simulink model "latest_coil"  (R2021b)
settings: Solver=FixedStepAuto  StartTime=-18e-3  StopTime=50e-3  FixedStep=1e-4  RelTol=1e-3
undefined symbols (not defined in the file): X, Y, Z
libraries: sm_lib x28, nesl_utility x9
(part 3 of 5)

== matlab function latest_coil/Inner Coil/Coil 1/FIELD Y ==
  data: X input; Hx_yp output; Y input; Z input; I input; Hy_yp output; Hz_yp output; Hx_yn output; Hy_yn output; Hz_yn output; dBx_dx output; dBx_dy output; dBx_dz output; dBz_dx output; dBz_dy output; dBz_dz output
function [Hx_yp, Hy_yp, Hz_yp, Hx_yn, Hy_yn, Hz_yn, dBx_dx, dBx_dy, dBx_dz, dBz_dx, dBz_dy, dBz_dz] = field_y(X, Y, Z, I)

n = 1;
gy = 520e-6;
% gx = 675e-6;
gz = 0;
m0 = 4*pi*1e-7;
k = 0.4e-3;
yp1 = -0.6e-3 - (n-1)*k;
yp2 = 0.6e-3 + (n-1)*k;
a_xp = gy;
a_zp = gz;
k_yp = 1./(4*pi*((a_xp-X).^2+(a_zp-Z).^2));
kyp = (yp2-Y)./((yp2-Y).^2+(a_xp-X).^2+(a_zp-Z).^2).^0.5;
k_2yp = (yp1-Y)./((yp1-Y).^2+(a_xp-X).^2+(a_zp-Z).^2).^0.5;

Hx_yp = -((a_zp-Z).*k_yp.*(kyp - k_2yp))*I*m0;
Hy_yp = zeros(size(X,1),size(Y,1),size(Z,1));
Hz_yp = (-(a_xp-X).*k_yp.*(kyp - k_2yp))*I*m0;

a_xn = -gy;
yn1 = -0.8e-3 - (n-1)*k;
yn2 = 0.8e-3 + (n-1)*k;
k_yn = 1./(4*pi*((a_xn-X).^2+(a_zp-Z).^2));
kyn = (yn2-Y)./((yn2-Y).^2+(a_xn-X).^2+(a_zp-Z).^2).^0.5;
k_2yn = (yn1-Y)./((yn1-Y).^2+(a_xn-X).^2+(a_zp-Z).^2).^0.5;

Hx_yn = ((a_zp-Z).*k_yn.*(kyn - k_2yn))*I*m0;
Hy_yn = zeros(size(X,1),size(Y,1),size(Z,1));
Hz_yn = ((a_xn-X).*k_yn.*(kyn - k_2yn))*I*m0;


dBxn_dx = - (I*Z*m0*(((Y - yn1)*(2*X - 2*a_xn))/(2*((X - a_xn)^2 + (Z - a_zp)^2 + (Y - yn1)^2)^(3/2)) - ((Y - yn2)*(2*X - 2*a_xn))/(2*((X - a_xn)^2 + (Z - a_zp)^2 + (Y - yn2)^2)^(3/2))))/(4*pi*((X - a_xn)^2 + (Z - a_zp)^2)) - (I*Z*m0*((Y - yn1)/((X - a_xn)^2 + (Z - a_zp)^2 + (Y - yn1)^2)^(1/2) - (Y - yn2)/((X - a_xn)^2 + (Z - a_zp)^2 + (Y - yn2)^2)^(1/2))*(2*X - 2*a_xn))/(4*pi*((X - a_xn)^2 + (Z - a_zp)^2)^2);
dBxp_dx = (I*Z*m0*(((Y - yp1)*(2*X - 2*a_xp))/(2*((X - a_xp)^2 + (Z - a_zp)^2 + (Y - yp1)^2)^(3/2)) - ((Y - yp2)*(2*X - 2*a_xp))/(2*((X - a_xp)^2 + (Z - a_zp)^2 + (Y - yp2)^2)^(3/2))))/(4*pi*((X - a_xp)^2 + (Z - a_zp)^2)) + (I*Z*m0*((Y - yp1)/((X - a_xp)^2 + (Z - a_zp)^2 + (Y - yp1)^2)^(1/2) - (Y - yp2)/((X - a_xp)^2 + (Z - a_zp)^2 + (Y - yp2)^2)^(1/2))*(2*X - 2*a_xp))/(4*pi*((X - a_xp)^2 + (Z - a_zp)^2)^2);
dBx_dx = dBxp_dx + dBxn_dx;

dBxp_dy = -(I*Z*m0*(1/((X - a_xp)^2 + (Z - a_zp)^2 + (Y - yp1)^2)^(1/2) - 1/((X - a_xp)^2 + (Z - a_zp)^2 + (Y - yp2)^2)^(1/2) - ((Y - yp1)*(2*Y - 2*yp1))/(2*((X - a_xp)^2 + (Z - a_zp)^2 + (Y - yp1)^2)^(3/2)) + ((Y - yp2)*(2*Y - 2*yp2))/(2*((X - a_xp)^2 + (Z - a_zp)^2 + (Y - yp2)^2)^(3/2))))/(4*pi*((X - a_xp)^2 + (Z - a_zp)^2));
dBxn_dy = (I*Z*m0*(1/((X - a_xn)^2 + (Z - a_zp)^2 + (Y - yn1)^2)^(1/2) - 1/((X - a_xn)^2 + (Z - a_zp)^2 + (Y - yn2)^2)^(1/2) - ((Y - yn1)*(2*Y - 2*yn1))/(2*((X - a_xn)^2 + (Z - a_zp)^2 + (Y - yn1)^2)^(3/2)) + ((Y - yn2)*(2*Y - 2*yn2))/(2*((X - a_xn)^2 + (Z - a_zp)^2 + (Y - yn2)^2)^(3/2))))/(4*pi*((X - a_xn)^2 + (Z - a_zp)^2));
dBx_dy = dBxp_dy + dBxn_dy;

dBxp_dz = (I*Z*m0*(((Y - yp1)*(2*Z - 2*a_zp))/(2*((X - a_xp)^2 + (Z - a_zp)^2 + (Y - yp1)^2)^(3/2)) - ((Y - yp2)*(2*Z - 2*a_zp))/(2*((X - a_xp)^2 + (Z - a_zp)^2 + (Y - yp2)^2)^(3/2))))/(4*pi*((X - a_xp)^2 + (Z - a_zp)^2)) - (I*m0*((Y - yp1)/((X - a_xp)^2 + (Z - a_zp)^2 + (Y - yp1)^2)^(1/2) - (Y - yp2)/((X - a_xp)^2 + (Z - a_zp)^2 + (Y - yp2)^2)^(1/2)))/(4*pi*((X - a_xp)^2 + (Z - a_zp)^2)) + (I*Z*m0*((Y - yp1)/((X - a_xp)^2 + (Z - a_zp)^2 + (Y - yp1)^2)^(1/2) - (Y - yp2)/((X - a_xp)^2 + (Z - a_zp)^2 + (Y - yp2)^2)^(1/2))*(2*Z - 2*a_zp))/(4*pi*((X - a_xp)^2 + (Z - a_zp)^2)^2);
dBxn_dz = (I*m0*((Y - yn1)/((X - a_xn)^2 + (Z - a_zp)^2 + (Y - yn1)^2)^(1/2) - (Y - yn2)/((X - a_xn)^2 + (Z - a_zp)^2 + (Y - yn2)^2)^(1/2)))/(4*pi*((X - a_xn)^2 + (Z - a_zp)^2)) - (I*Z*m0*(((Y - yn1)*(2*Z - 2*a_zp))/(2*((X - a_xn)^2 + (Z - a_zp)^2 + (Y - yn1)^2)^(3/2)) - ((Y - yn2)*(2*Z - 2*a_zp))/(2*((X - a_xn)^2 + (Z - a_zp)^2 + (Y - yn2)^2)^(3/2))))/(4*pi*((X - a_xn)^2 + (Z - a_zp)^2)) - (I*Z*m0*((Y - yn1)/((X - a_xn)^2 + (Z - a_zp)^2 + (Y - yn1)^2)^(1/2) - (Y - yn2)/((X - a_xn)^2 + (Z - a_zp)^2 + (Y - yn2)^2)^(1/2))*(2*Z - 2*a_zp))/(4*pi*((X - a_xn)^2 + (Z - a_zp)^2)^2);
dBx_dz = dBxp_dz + dBxn_dz;

dBzn_dx = (I*m0*(X - a_xn)*(((Y - yn1)*(2*X - 2*a_xn))/(2*((X - a_xn)^2 + (Z - a_zp)^2 + (Y - yn1)^2)^(3/2)) - ((Y - yn2)*(2*X - 2*a_xn))/(2*((X - a_xn)^2 + (Z - a_zp)^2 + (Y - yn2)^2)^(3/2))))/(4*pi*(Z^2 + (X - a_xn)^2)) - (I*m0*((Y - yn1)/((X - a_xn)^2 + (Z - a_zp)^2 + (Y - yn1)^2)^(1/2) - (Y - yn2)/((X - a_xn)^2 + (Z - a_zp)^2 + (Y - yn2)^2)^(1/2)))/(4*pi*(Z^2 + (X - a_xn)^2)) + (I*m0*((Y - yn1)/((X - a_xn)^2 + (Z - a_zp)^2 + (Y - yn1)^2)^(1/2) - (Y - yn2)/((X - a_xn)^2 + (Z - a_zp)^2 + (Y - yn2)^2)^(1/2))*(X - a_xn)*(2*X - 2*a_xn))/(4*pi*(Z^2 + (X - a_xn)^2)^2);
dBzp_dx = (I*m0*((Y - yp1)/((X - a_xp)^2 + (Z - a_zp)^2 + (Y - yp1)^2)^(1/2) - (Y - yp2)/((X - a_xp)^2 + (Z - a_zp)^2 + (Y - yp2)^2)^(1/2)))/(4*pi*(Z^2 + (X - a_xp)^2)) - (I*m0*(X - a_xp)*(((Y - yp1)*(2*X - 2*a_xp))/(2*((X - a_xp)^2 + (Z - a_zp)^2 + (Y - yp1)^2)^(3/2)) - ((Y - yp2)*(2*X - 2*a_xp))/(2*((X - a_xp)^2 + (Z - a_zp)^2 + (Y - yp2)^2)^(3/2))))/(4*pi*(Z^2 + (X - a_xp)^2)) - (I*m0*((Y - yp1)/((X - a_xp)^2 + (Z - a_zp)^2 + (Y - yp1)^2)^(1/2) - (Y - yp2)/((X - a_xp)^2 + (Z - a_zp)^2 + (Y - yp2)^2)^(1/2))*(X - a_xp)*(2*X - 2*a_xp))/(4*pi*(Z^2 + (X - a_xp)^2)^2);
dBz_dx = dBzp_dx + dBzn_dx;

dBzn_dy = -(I*m0*(X - a_xn)*(1/((X - a_xn)^2 + (Z - a_zp)^2 + (Y - yn1)^2)^(1/2) - 1/((X - a_xn)^2 + (Z - a_zp)^2 + (Y - yn2)^2)^(1/2) - ((Y - yn1)*(2*Y - 2*yn1))/(2*((X - a_xn)^2 + (Z - a_zp)^2 + (Y - yn1)^2)^(3/2)) + ((Y - yn2)*(2*Y - 2*yn2))/(2*((X - a_xn)^2 + (Z - a_zp)^2 + (Y - yn2)^2)^(3/2))))/(4*pi*(Z^2 + (X - a_xn)^2));
dBzp_dy = (I*m0*(X - a_xp)*(1/((X - a_xp)^2 + (Z - a_zp)^2 + (Y - yp1)^2)^(1/2) - 1/((X - a_xp)^2 + (Z - a_zp)^2 + (Y - yp2)^2)^(1/2) - ((Y - yp1)*(2*Y - 2*yp1))/(2*((X - a_xp)^2 + (Z - a_zp)^2 + (Y - yp1)^2)^(3/2)) + ((Y - yp2)*(2*Y - 2*yp2))/(2*((X - a_xp)^2 + (Z - a_zp)^2 + (Y - yp2)^2)^(3/2))))/(4*pi*(Z^2 + (X - a_xp)^2));
dBz_dy = dBzn_dy + dBzp_dy;

dBzn_dz = (I*m0*(X - a_xn)*(((Y - yn1)*(2*Z - 2*a_zp))/(2*((X - a_xn)^2 + (Z - a_zp)^2 + (Y - yn1)^2)^(3/2)) - ((Y - yn2)*(2*Z - 2*a_zp))/(2*((X - a_xn)^2 + (Z - a_zp)^2 + (Y - yn2)^2)^(3/2))))/(4*pi*(Z^2 + (X - a_xn)^2)) + (I*Z*m0*((Y - yn1)/((X - a_xn)^2 + (Z - a_zp)^2 + (Y - yn1)^2)^(1/2) - (Y - yn2)/((X - a_xn)^2 + (Z - a_zp)^2 + (Y - yn2)^2)^(1/2))*(X - a_xn))/(2*pi*(Z^2 + (X - a_xn)^2)^2);
dBzp_dz = - (I*m0*(X - a_xp)*(((Y - yp1)*(2*Z - 2*a_zp))/(2*((X - a_xp)^2 + (Z - a_zp)^2 + (Y - yp1)^2)^(3/2)) - ((Y - yp2)*(2*Z - 2*a_zp))/(2*((X - a_xp)^2 + (Z - a_zp)^2 + (Y - yp2)^2)^(3/2))))/(4*pi*(Z^2 + (X - a_xp)^2)) - (I*Z*m0*((Y - yp1)/((X - a_xp)^2 + (Z - a_zp)^2 + (Y - yp1)^2)^(1/2) - (Y - yp2)/((X - a_xp)^2 + (Z - a_zp)^2 + (Y - yp2)^2)^(1/2))*(X - a_xp))/(2*pi*(Z^2 + (X - a_xp)^2)^2);
dBz_dz = dBzn_dz + dBzp_dz;
end

== matlab function latest_coil/Inner Coil/Coil 5/MATLAB Function ==
  data: X input; Hx_xp output; Y input; Z input; I input; Hy_xp output; Hz_xp output; Hx_xn output; Hy_xn output; Hz_xn output; dBy_dx output; dBy_dy output; dBy_dz output; dBz_dx output; dBz_dy output; dBz_dz output
function [Hx_xp, Hy_xp, Hz_xp, Hx_xn, Hy_xn, Hz_xn,dBy_dx ,dBy_dy, dBy_dz, dBz_dx ,dBz_dy, dBz_dz] = field_x(X, Y, Z, I)
n = 5;
gy = 424e-6;
gx = 2.275e-3;
gz = 0;
m0 = 4*pi*1e-7;
k = 0.4e-3;
xp1 = -0.8e-3 - (n-1)*k;
xp2 = 0.8e-3 + (n-1)*k;
a_yp = gx; 
a_zp = gz;
k_p = 1./(4*pi*((a_yp-Y).^2+(a_zp-Z).^2));
kxp = (xp2-X)./((xp2-X).^2+(a_yp-Y).^2+(a_zp-Z).^2).^0.5;
k_2xp = (xp1-X)./((xp1-X).^2+(a_yp-Y).^2+(a_zp-Z).^2).^0.5;

Hx_xp = zeros(size(X,1),size(Y,1),size(Z,1));
Hy_xp = (-(a_zp-Z).*k_p.*(kxp - k_2xp))*I*m0;
Hz_xp = (-(a_yp-Y).*k_p.*(kxp - k_2xp))*I*m0;

a_yn = -gx;
xn1 = -1e-3 - (n-1)*k;
xn2 = 1e-3 + (n-1)*k;
k_n = 1./(4*pi*((a_yn-Y).^2+(a_zp-Z).^2));
kxn = (xn2-X)./((xn2-X).^2+(a_yn-Y).^2+(a_zp-Z).^2).^0.5;
k_2xn = (xn1-X)./((xn1-X).^2+(a_yn-Y).^2+(a_zp-Z).^2).^0.5;

Hx_xn = zeros(size(X,1),size(Y,1),size(Z,1));
Hy_xn = ((a_zp-Z).*k_n.*(kxn - k_2xn))*I*m0;
Hz_xn = ((a_yn-Y).*k_n.*(kxn - k_2xn))*I*m0;

dByn_dx = (I*Z*m0*(1/((Y - a_yn)^2 + (Z - a_zp)^2 + (X - xn1)^2)^(1/2) - 1/((Y - a_yn)^2 + (Z - a_zp)^2 + (X - xn2)^2)^(1/2) - ((X - xn1)*(2*X - 2*xn1))/(2*((Y - a_yn)^2 + (Z - a_zp)^2 + (X - xn1)^2)^(3/2)) + ((X - xn2)*(2*X - 2*xn2))/(2*((Y - a_yn)^2 + (Z - a_zp)^2 + (X - xn2)^2)^(3/2))))/(4*pi*((Y - a_yn)^2 + (Z - a_zp)^2));
dByp_dx = -(I*Z*m0*(1/((Y - a_yp)^2 + (Z - a_zp)^2 + (X - xp1)^2)^(1/2) - 1/((Y - a_yp)^2 + (Z - a_zp)^2 + (X - xp2)^2)^(1/2) - ((X - xp1)*(2*X - 2*xp1))/(2*((Y - a_yp)^2 + (Z - a_zp)^2 + (X - xp1)^2)^(3/2)) + ((X - xp2)*(2*X - 2*xp2))/(2*((Y - a_yp)^2 + (Z - a_zp)^2 + (X - xp2)^2)^(3/2))))/(4*pi*((Y - a_yp)^2 + (Z - a_zp)^2));
dBy_dx = dByp_dx + dByn_dx;

dByp_dy = (I*Z*m0*(((X - xp1)*(2*Y - 2*a_yp))/(2*((Y - a_yp)^2 + (Z - a_zp)^2 + (X - xp1)^2)^(3/2)) - ((X - xp2)*(2*Y - 2*a_yp))/(2*((Y - a_yp)^2 + (Z - a_zp)^2 + (X - xp2)^2)^(3/2))))/(4*pi*((Y - a_yp)^2 + (Z - a_zp)^2)) + (I*Z*m0*(2*Y - 2*a_yp)*((X - xp1)/((Y - a_yp)^2 + (Z - a_zp)^2 + (X - xp1)^2)^(1/2) - (X - xp2)/((Y - a_yp)^2 + (Z - a_zp)^2 + (X - xp2)^2)^(1/2)))/(4*pi*((Y - a_yp)^2 + (Z - a_zp)^2)^2);
dByn_dy = - (I*Z*m0*(((X - xn1)*(2*Y - 2*a_yn))/(2*((Y - a_yn)^2 + (Z - a_zp)^2 + (X - xn1)^2)^(3/2)) - ((X - xn2)*(2*Y - 2*a_yn))/(2*((Y - a_yn)^2 + (Z - a_zp)^2 + (X - xn2)^2)^(3/2))))/(4*pi*((Y - a_yn)^2 + (Z - a_zp)^2)) - (I*Z*m0*(2*Y - 2*a_yn)*((X - xn1)/((Y - a_yn)^2 + (Z - a_zp)^2 + (X - xn1)^2)^(1/2) - (X - xn2)/((Y - a_yn)^2 + (Z - a_zp)^2 + (X - xn2)^2)^(1/2)))/(4*pi*((Y - a_yn)^2 + (Z - a_zp)^2)^2);
dBy_dy = dByp_dy + dByn_dy;

dByp_dz = (I*Z*m0*(((X - xp1)*(2*Z - 2*a_zp))/(2*((Y - a_yp)^2 + (Z - a_zp)^2 + (X - xp1)^2)^(3/2)) - ((X - xp2)*(2*Z - 2*a_zp))/(2*((Y - a_yp)^2 + (Z - a_zp)^2 + (X - xp2)^2)^(3/2))))/(4*pi*((Y - a_yp)^2 + (Z - a_zp)^2)) - (I*m0*((X - xp1)/((Y - a_yp)^2 + (Z - a_zp)^2 + (X - xp1)^2)^(1/2) - (X - xp2)/((Y - a_yp)^2 + (Z - a_zp)^2 + (X - xp2)^2)^(1/2)))/(4*pi*((Y - a_yp)^2 + (Z - a_zp)^2)) + (I*Z*m0*(2*Z - 2*a_zp)*((X - xp1)/((Y - a_yp)^2 + (Z - a_zp)^2 + (X - xp1)^2)^(1/2) - (X - xp2)/((Y - a_yp)^2 + (Z - a_zp)^2 + (X - xp2)^2)^(1/2)))/(4*pi*((Y - a_yp)^2 + (Z - a_zp)^2)^2);
dByn_dz = (I*m0*((X - xn1)/((Y - a_yn)^2 + (Z - a_zp)^2 + (X - xn1)^2)^(1/2) - (X - xn2)/((Y - a_yn)^2 + (Z - a_zp)^2 + (X - xn2)^2)^(1/2)))/(4*pi*((Y - a_yn)^2 + (Z - a_zp)^2)) - (I*Z*m0*(((X - xn1)*(2*Z - 2*a_zp))/(2*((Y - a_yn)^2 + (Z - a_zp)^2 + (X - xn1)^2)^(3/2)) - ((X - xn2)*(2*Z - 2*a_zp))/(2*((Y - a_yn)^2 + (Z - a_zp)^2 + (X - xn2)^2)^(3/2))))/(4*pi*((Y - a_yn)^2 + (Z - a_zp)^2)) - (I*Z*m0*(2*Z - 2*a_zp)*((X - xn1)/((Y - a_yn)^2 + (Z - a_zp)^2 + (X - xn1)^2)^(1/2) - (X - xn2)/((Y - a_yn)^2 + (Z - a_zp)^2 + (X - xn2)^2)^(1/2)))/(4*pi*((Y - a_yn)^2 + (Z - a_zp)^2)^2);
dBy_dz = dByp_dz + dByn_dz;

dBzp_dx = (I*m0*(Y - a_yp)*(1/((Y - a_yp)^2 + (Z - a_zp)^2 + (X - xp1)^2)^(1/2) - 1/((Y - a_yp)^2 + (Z - a_zp)^2 + (X - xp2)^2)^(1/2) - ((X - xp1)*(2*X - 2*xp1))/(2*((Y - a_yp)^2 + (Z - a_zp)^2 + (X - xp1)^2)^(3/2)) + ((X - xp2)*(2*X - 2*xp2))/(2*((Y - a_yp)^2 + (Z - a_zp)^2 + (X - xp2)^2)^(3/2))))/(4*pi*(Z^2 + (Y - a_yp)^2));
dBzn_dx = -(I*m0*(Y - a_yn)*(1/((Y - a_yn)^2 + (Z - a_zp)^2 + (X - xn1)^2)^(1/2) - 1/((Y - a_yn)^2 + (Z - a_zp)^2 + (X - xn2)^2)^(1/2) - ((X - xn1)*(2*X - 2*xn1))/(2*((Y - a_yn)^2 + (Z - a_zp)^2 + (X - xn1)^2)^(3/2)) + ((X - xn2)*(2*X - 2*xn2))/(2*((Y - a_yn)^2 + (Z - a_zp)^2 + (X - xn2)^2)^(3/2))))/(4*pi*(Z^2 + (Y - a_yn)^2));
dBz_dx = dBzp_dx + dBzn_dx;

dBzn_dy = (I*m0*(Y - a_yn)*(((X - xn1)*(2*Y - 2*a_yn))/(2*((Y - a_yn)^2 + (Z - a_zp)^2 + (X - xn1)^2)^(3/2)) - ((X - xn2)*(2*Y - 2*a_yn))/(2*((Y - a_yn)^2 + (Z - a_zp)^2 + (X - xn2)^2)^(3/2))))/(4*pi*(Z^2 + (Y - a_yn)^2)) - (I*m0*((X - xn1)/((Y - a_yn)^2 + (Z - a_zp)^2 + (X - xn1)^2)^(1/2) - (X - xn2)/((Y - a_yn)^2 + (Z - a_zp)^2 + (X - xn2)^2)^(1/2)))/(4*pi*(Z^2 + (Y - a_yn)^2)) + (I*m0*(Y - a_yn)*(2*Y - 2*a_yn)*((X - xn1)/((Y - a_yn)^2 + (Z - a_zp)^2 + (X - xn1)^2)^(1/2) - (X - xn2)/((Y - a_yn)^2 + (Z - a_zp)^2 + (X - xn2)^2)^(1/2)))/(4*pi*(Z^2 + (Y - a_yn)^2)^2);
dBzp_dy = (I*m0*((X - xp1)/((Y - a_yp)^2 + (Z - a_zp)^2 + (X - xp1)^2)^(1/2) - (X - xp2)/((Y - a_yp)^2 + (Z - a_zp)^2 + (X - xp2)^2)^(1/2)))/(4*pi*(Z^2 + (Y - a_yp)^2)) - (I*m0*(Y - a_yp)*(((X - xp1)*(2*Y - 2*a_yp))/(2*((Y - a_yp)^2 + (Z - a_zp)^2 + (X - xp1)^2)^(3/2)) - ((X - xp2)*(2*Y - 2*a_yp))/(2*((Y - a_yp)^2 + (Z - a_zp)^2 + (X - xp2)^2)^(3/2))))/(4*pi*(Z^2 + (Y - a_yp)^2)) - (I*m0*(Y - a_yp)*(2*Y - 2*a_yp)*((X - xp1)/((Y - a_yp)^2 + (Z - a_zp)^2 + (X - xp1)^2)^(1/2) - (X - xp2)/((Y - a_yp)^2 + (Z - a_zp)^2 + (X - xp2)^2)^(1/2)))/(4*pi*(Z^2 + (Y - a_yp)^2)^2);
dBz_dy = dBzn_dy + dBzp_dy;

dBzn_dz = (I*m0*(Y - a_yn)*(((X - xn1)*(2*Z - 2*a_zp))/(2*((Y - a_yn)^2 + (Z - a_zp)^2 + (X - xn1)^2)^(3/2)) - ((X - xn2)*(2*Z - 2*a_zp))/(2*((Y - a_yn)^2 + (Z - a_zp)^2 + (X - xn2)^2)^(3/2))))/(4*pi*(Z^2 + (Y - a_yn)^2)) + (I*Z*m0*(Y - a_yn)*((X - xn1)/((Y - a_yn)^2 + (Z - a_zp)^2 + (X - xn1)^2)^(1/2) - (X - xn2)/((Y - a_yn)^2 + (Z - a_zp)^2 + (X - xn2)^2)^(1/2)))/(2*pi*(Z^2 + (Y - a_yn)^2)^2);
dBzp_dz = - (I*m0*(Y - a_yp)*(((X - xp1)*(2*Z - 2*a_zp))/(2*((Y - a_yp)^2 + (Z - a_zp)^2 + (X - xp1)^2)^(3/2)) - ((X - xp2)*(2*Z - 2*a_zp))/(2*((Y - a_yp)^2 + (Z - a_zp)^2 + (X - xp2)^2)^(3/2))))/(4*pi*(Z^2 + (Y - a_yp)^2)) - (I*Z*m0*(Y - a_yp)*((X - xp1)/((Y - a_yp)^2 + (Z - a_zp)^2 + (X - xp1)^2)^(1/2) - (X - xp2)/((Y - a_yp)^2 + (Z - a_zp)^2 + (X - xp2)^2)^(1/2)))/(2*pi*(Z^2 + (Y - a_yp)^2)^2);
dBz_dz = dBzn_dz + dBzp_dz;
end

== matlab function latest_coil/Inner Coil/Coil 5/MATLAB Function3 ==
  data: X input; Hx_yp output; Y input; Z input; I input; Hy_yp output; Hz_yp output; Hx_yn output; Hy_yn output; Hz_yn output; dBx_dx output; dBx_dy output; dBx_dz output; dBz_dx output; dBz_dy output; dBz_dz output
function [Hx_yp, Hy_yp, Hz_yp, Hx_yn, Hy_yn, Hz_yn, dBx_dx, dBx_dy, dBx_dz, dBz_dx, dBz_dy, dBz_dz] = field_y(X, Y, Z, I)
n = 5;
gy = 424e-6;
gx = 2.275e-3;
gz = 0;
m0 = 4*pi*1e-7;
k = 0.4e-3;
yp1 = -0.6e-3 - (n-1)*k;
yp2 = 0.6e-3 + (n-1)*k;
a_xp = gy;
a_zp = gz;
k_yp = 1./(4*pi*((a_xp-X).^2+(a_zp-Z).^2));
kyp = (yp2-Y)./((yp2-Y).^2+(a_xp-X).^2+(a_zp-Z).^2).^0.5;
k_2yp = (yp1-Y)./((yp1-Y).^2+(a_xp-X).^2+(a_zp-Z).^2).^0.5;

Hx_yp = -((a_zp-Z).*k_yp.*(kyp - k_2yp))*I*m0;
Hy_yp = zeros(size(X,1),size(Y,1),size(Z,1));
Hz_yp = (-(a_xp-X).*k_yp.*(kyp - k_2yp))*I*m0;

a_xn = -gy;
yn1 = -0.8e-3 - (n-1)*k;
yn2 = 0.8e-3 + (n-1)*k;
k_yn = 1./(4*pi*((a_xn-X).^2+(a_zp-Z).^2));
kyn = (yn2-Y)./((yn2-Y).^2+(a_xn-X).^2+(a_zp-Z).^2).^0.5;
k_2yn = (yn1-Y)./((yn1-Y).^2+(a_xn-X).^2+(a_zp-Z).^2).^0.5;

Hx_yn = ((a_zp-Z).*k_yn.*(kyn - k_2yn))*I*m0;
Hy_yn = zeros(size(X,1),size(Y,1),size(Z,1));
Hz_yn = ((a_xn-X).*k_yn.*(kyn - k_2yn))*I*m0;

dBxn_dx = - (I*Z*m0*(((Y - yn1)*(2*X - 2*a_xn))/(2*((X - a_xn)^2 + (Z - a_zp)^2 + (Y - yn1)^2)^(3/2)) - ((Y - yn2)*(2*X - 2*a_xn))/(2*((X - a_xn)^2 + (Z - a_zp)^2 + (Y - yn2)^2)^(3/2))))/(4*pi*((X - a_xn)^2 + (Z - a_zp)^2)) - (I*Z*m0*((Y - yn1)/((X - a_xn)^2 + (Z - a_zp)^2 + (Y - yn1)^2)^(1/2) - (Y - yn2)/((X - a_xn)^2 + (Z - a_zp)^2 + (Y - yn2)^2)^(1/2))*(2*X - 2*a_xn))/(4*pi*((X - a_xn)^2 + (Z - a_zp)^2)^2);
dBxp_dx = (I*Z*m0*(((Y - yp1)*(2*X - 2*a_xp))/(2*((X - a_xp)^2 + (Z - a_zp)^2 + (Y - yp1)^2)^(3/2)) - ((Y - yp2)*(2*X - 2*a_xp))/(2*((X - a_xp)^2 + (Z - a_zp)^2 + (Y - yp2)^2)^(3/2))))/(4*pi*((X - a_xp)^2 + (Z - a_zp)^2)) + (I*Z*m0*((Y - yp1)/((X - a_xp)^2 + (Z - a_zp)^2 + (Y - yp1)^2)^(1/2) - (Y - yp2)/((X - a_xp)^2 + (Z - a_zp)^2 + (Y - yp2)^2)^(1/2))*(2*X - 2*a_xp))/(4*pi*((X - a_xp)^2 + (Z - a_zp)^2)^2);
dBx_dx = dBxp_dx + dBxn_dx;

dBxp_dy = -(I*Z*m0*(1/((X - a_xp)^2 + (Z - a_zp)^2 + (Y - yp1)^2)^(1/2) - 1/((X - a_xp)^2 + (Z - a_zp)^2 + (Y - yp2)^2)^(1/2) - ((Y - yp1)*(2*Y - 2*yp1))/(2*((X - a_xp)^2 + (Z - a_zp)^2 + (Y - yp1)^2)^(3/2)) + ((Y - yp2)*(2*Y - 2*yp2))/(2*((X - a_xp)^2 + (Z - a_zp)^2 + (Y - yp2)^2)^(3/2))))/(4*pi*((X - a_xp)^2 + (Z - a_zp)^2));
dBxn_dy = (I*Z*m0*(1/((X - a_xn)^2 + (Z - a_zp)^2 + (Y - yn1)^2)^(1/2) - 1/((X - a_xn)^2 + (Z - a_zp)^2 + (Y - yn2)^2)^(1/2) - ((Y - yn1)*(2*Y - 2*yn1))/(2*((X - a_xn)^2 + (Z - a_zp)^2 + (Y - yn1)^2)^(3/2)) + ((Y - yn2)*(2*Y - 2*yn2))/(2*((X - a_xn)^2 + (Z - a_zp)^2 + (Y - yn2)^2)^(3/2))))/(4*pi*((X - a_xn)^2 + (Z - a_zp)^2));
dBx_dy = dBxp_dy + dBxn_dy;

dBxp_dz = (I*Z*m0*(((Y - yp1)*(2*Z - 2*a_zp))/(2*((X - a_xp)^2 + (Z - a_zp)^2 + (Y - yp1)^2)^(3/2)) - ((Y - yp2)*(2*Z - 2*a_zp))/(2*((X - a_xp)^2 + (Z - a_zp)^2 + (Y - yp2)^2)^(3/2))))/(4*pi*((X - a_xp)^2 + (Z - a_zp)^2)) - (I*m0*((Y - yp1)/((X - a_xp)^2 + (Z - a_zp)^2 + (Y - yp1)^2)^(1/2) - (Y - yp2)/((X - a_xp)^2 + (Z - a_zp)^2 + (Y - yp2)^2)^(1/2)))/(4*pi*((X - a_xp)^2 + (Z - a_zp)^2)) + (I*Z*m0*((Y - yp1)/((X - a_xp)^2 + (Z - a_zp)^2 + (Y - yp1)^2)^(1/2) - (Y - yp2)/((X - a_xp)^2 + (Z - a_zp)^2 + (Y - yp2)^2)^(1/2))*(2*Z - 2*a_zp))/(4*pi*((X - a_xp)^2 + (Z - a_zp)^2)^2);
dBxn_dz = (I*m0*((Y - yn1)/((X - a_xn)^2 + (Z - a_zp)^2 + (Y - yn1)^2)^(1/2) - (Y - yn2)/((X - a_xn)^2 + (Z - a_zp)^2 + (Y - yn2)^2)^(1/2)))/(4*pi*((X - a_xn)^2 + (Z - a_zp)^2)) - (I*Z*m0*(((Y - yn1)*(2*Z - 2*a_zp))/(2*((X - a_xn)^2 + (Z - a_zp)^2 + (Y - yn1)^2)^(3/2)) - ((Y - yn2)*(2*Z - 2*a_zp))/(2*((X - a_xn)^2 + (Z - a_zp)^2 + (Y - yn2)^2)^(3/2))))/(4*pi*((X - a_xn)^2 + (Z - a_zp)^2)) - (I*Z*m0*((Y - yn1)/((X - a_xn)^2 + (Z - a_zp)^2 + (Y - yn1)^2)^(1/2) - (Y - yn2)/((X - a_xn)^2 + (Z - a_zp)^2 + (Y - yn2)^2)^(1/2))*(2*Z - 2*a_zp))/(4*pi*((X - a_xn)^2 + (Z - a_zp)^2)^2);
dBx_dz = dBxp_dz + dBxn_dz;

dBzn_dx = (I*m0*(X - a_xn)*(((Y - yn1)*(2*X - 2*a_xn))/(2*((X - a_xn)^2 + (Z - a_zp)^2 + (Y - yn1)^2)^(3/2)) - ((Y - yn2)*(2*X - 2*a_xn))/(2*((X - a_xn)^2 + (Z - a_zp)^2 + (Y - yn2)^2)^(3/2))))/(4*pi*(Z^2 + (X - a_xn)^2)) - (I*m0*((Y - yn1)/((X - a_xn)^2 + (Z - a_zp)^2 + (Y - yn1)^2)^(1/2) - (Y - yn2)/((X - a_xn)^2 + (Z - a_zp)^2 + (Y - yn2)^2)^(1/2)))/(4*pi*(Z^2 + (X - a_xn)^2)) + (I*m0*((Y - yn1)/((X - a_xn)^2 + (Z - a_zp)^2 + (Y - yn1)^2)^(1/2) - (Y - yn2)/((X - a_xn)^2 + (Z - a_zp)^2 + (Y - yn2)^2)^(1/2))*(X - a_xn)*(2*X - 2*a_xn))/(4*pi*(Z^2 + (X - a_xn)^2)^2);
dBzp_dx = (I*m0*((Y - yp1)/((X - a_xp)^2 + (Z - a_zp)^2 + (Y - yp1)^2)^(1/2) - (Y - yp2)/((X - a_xp)^2 + (Z - a_zp)^2 + (Y - yp2)^2)^(1/2)))/(4*pi*(Z^2 + (X - a_xp)^2)) - (I*m0*(X - a_xp)*(((Y - yp1)*(2*X - 2*a_xp))/(2*((X - a_xp)^2 + (Z - a_zp)^2 + (Y - yp1)^2)^(3/2)) - ((Y - yp2)*(2*X - 2*a_xp))/(2*((X - a_xp)^2 + (Z - a_zp)^2 + (Y - yp2)^2)^(3/2))))/(4*pi*(Z^2 + (X - a_xp)^2)) - (I*m0*((Y - yp1)/((X - a_xp)^2 + (Z - a_zp)^2 + (Y - yp1)^2)^(1/2) - (Y - yp2)/((X - a_xp)^2 + (Z - a_zp)^2 + (Y - yp2)^2)^(1/2))*(X - a_xp)*(2*X - 2*a_xp))/(4*pi*(Z^2 + (X - a_xp)^2)^2);
dBz_dx = dBzp_dx + dBzn_dx;

dBzn_dy = -(I*m0*(X - a_xn)*(1/((X - a_xn)^2 + (Z - a_zp)^2 + (Y - yn1)^2)^(1/2) - 1/((X - a_xn)^2 + (Z - a_zp)^2 + (Y - yn2)^2)^(1/2) - ((Y - yn1)*(2*Y - 2*yn1))/(2*((X - a_xn)^2 + (Z - a_zp)^2 + (Y - yn1)^2)^(3/2)) + ((Y - yn2)*(2*Y - 2*yn2))/(2*((X - a_xn)^2 + (Z - a_zp)^2 + (Y - yn2)^2)^(3/2))))/(4*pi*(Z^2 + (X - a_xn)^2));
dBzp_dy = (I*m0*(X - a_xp)*(1/((X - a_xp)^2 + (Z - a_zp)^2 + (Y - yp1)^2)^(1/2) - 1/((X - a_xp)^2 + (Z - a_zp)^2 + (Y - yp2)^2)^(1/2) - ((Y - yp1)*(2*Y - 2*yp1))/(2*((X - a_xp)^2 + (Z - a_zp)^2 + (Y - yp1)^2)^(3/2)) + ((Y - yp2)*(2*Y - 2*yp2))/(2*((X - a_xp)^2 + (Z - a_zp)^2 + (Y - yp2)^2)^(3/2))))/(4*pi*(Z^2 + (X - a_xp)^2));
dBz_dy = dBzn_dy + dBzp_dy;

dBzn_dz = (I*m0*(X - a_xn)*(((Y - yn1)*(2*Z - 2*a_zp))/(2*((X - a_xn)^2 + (Z - a_zp)^2 + (Y - yn1)^2)^(3/2)) - ((Y - yn2)*(2*Z - 2*a_zp))/(2*((X - a_xn)^2 + (Z - a_zp)^2 + (Y - yn2)^2)^(3/2))))/(4*pi*(Z^2 + (X - a_xn)^2)) + (I*Z*m0*((Y - yn1)/((X - a_xn)^2 + (Z - a_zp)^2 + (Y - yn1)^2)^(1/2) - (Y - yn2)/((X - a_xn)^2 + (Z - a_zp)^2 + (Y - yn2)^2)^(1/2))*(X - a_xn))/(2*pi*(Z^2 + (X - a_xn)^2)^2);
dBzp_dz = - (I*m0*(X - a_xp)*(((Y - yp1)*(2*Z - 2*a_zp))/(2*((X - a_xp)^2 + (Z - a_zp)^2 + (Y - yp1)^2)^(3/2)) - ((Y - yp2)*(2*Z - 2*a_zp))/(2*((X - a_xp)^2 + (Z - a_zp)^2 + (Y - yp2)^2)^(3/2))))/(4*pi*(Z^2 + (X - a_xp)^2)) - (I*Z*m0*((Y - yp1)/((X - a_xp)^2 + (Z - a_zp)^2 + (Y - yp1)^2)^(1/2) - (Y - yp2)/((X - a_xp)^2 + (Z - a_zp)^2 + (Y - yp2)^2)^(1/2))*(X - a_xp))/(2*pi*(Z^2 + (X - a_xp)^2)^2);
dBz_dz = dBzn_dz + dBzp_dz;
end

== matlab function latest_coil/Inner Coil/Coil 5/MATLAB Function4 ==
  data: Hx_xp input; Hy_xp input; Hz_xp input; Hx output; Hx_xn input; Hy_xn input; Hy output; Hz output; Hz_xn input; Hx_yp input; Hy_yp input; Hz_yp input; Hx_yn input; Hy_yn input; Hz_yn input
function [Hx, Hy, Hz] = field_sum(Hx_xp, Hy_xp, Hz_xp, Hx_xn, Hy_xn, Hz_xn, Hx_yp, Hy_yp, Hz_yp, Hx_yn, Hy_yn, Hz_yn)
Hx = Hx_xp + Hx_xn + Hx_yp + Hx_yn;
Hy = Hy_xp + Hy_xn + Hy_yp + Hy_yn;
Hz = Hz_xp + Hz_xn + Hz_yp + Hz_yn;
end

== matlab function latest_coil/Outer Coil/Coil 6/MATLAB Function ==
  data: X input; Hx_xp output; Y input; Z input; I input; Hy_xp output; Hz_xp output; Hx_xn output; Hy_xn output; Hz_xn output; dBy_dx output; dBy_dy output; dBy_dz output; dBz_dx output; dBz_dy output; dBz_dz output
function [Hx_xp, Hy_xp, Hz_xp, Hx_xn, Hy_xn, Hz_xn,dBy_dx ,dBy_dy, dBy_dz, dBz_dx ,dBz_dy, dBz_dz] = field_x(X, Y, Z, I)
n = 6;
% gy = 420e-6;
gx = 2.675e-3; 
gz = 0;
m0 = 4*pi*1e-7;
k = 0.4e-3;
xp1 = -0.8e-3 - (n-1)*k;
xp2 = 0.8e-3 + (n-1)*k;
a_yp = gx; 
a_zp = gz;
k_p = 1./(4*pi*((a_yp-Y).^2+(a_zp-Z).^2));
kxp = (xp2-X)./((xp2-X).^2+(a_yp-Y).^2+(a_zp-Z).^2).^0.5;
k_2xp = (xp1-X)./((xp1-X).^2+(a_yp-Y).^2+(a_zp-Z).^2).^0.5;

Hx_xp = zeros(size(X,1),size(Y,1),size(Z,1));
Hy_xp = (-(a_zp-Z).*k_p.*(kxp - k_2xp))*I*m0;
Hz_xp = (-(a_yp-Y).*k_p.*(kxp - k_2xp))*I*m0;

a_yn = -gx;
xn1 = -1e-3 - (n-1)*k;
xn2 = 1e-3 + (n-1)*k;
k_n = 1./(4*pi*((a_yn-Y).^2+(a_zp-Z).^2));
kxn = (xn2-X)./((xn2-X).^2+(a_yn-Y).^2+(a_zp-Z).^2).^0.5;
k_2xn = (xn1-X)./((xn1-X).^2+(a_yn-Y).^2+(a_zp-Z).^2).^0.5;

Hx_xn = zeros(size(X,1),size(Y,1),size(Z,1));
Hy_xn = ((a_zp-Z).*k_n.*(kxn - k_2xn))*I*m0;
Hz_xn = ((a_yn-Y).*k_n.*(kxn - k_2xn))*I*m0;
dByn_dx = (I*Z*m0*(1/((Y - a_yn)^2 + (Z - a_zp)^2 + (X - xn1)^2)^(1/2) - 1/((Y - a_yn)^2 + (Z - a_zp)^2 + (X - xn2)^2)^(1/2) - ((X - xn1)*(2*X - 2*xn1))/(2*((Y - a_yn)^2 + (Z - a_zp)^2 + (X - xn1)^2)^(3/2)) + ((X - xn2)*(2*X - 2*xn2))/(2*((Y - a_yn)^2 + (Z - a_zp)^2 + (X - xn2)^2)^(3/2))))/(4*pi*((Y - a_yn)^2 + (Z - a_zp)^2));
dByp_dx = -(I*Z*m0*(1/((Y - a_yp)^2 + (Z - a_zp)^2 + (X - xp1)^2)^(1/2) - 1/((Y - a_yp)^2 + (Z - a_zp)^2 + (X - xp2)^2)^(1/2) - ((X - xp1)*(2*X - 2*xp1))/(2*((Y - a_yp)^2 + (Z - a_zp)^2 + (X - xp1)^2)^(3/2)) + ((X - xp2)*(2*X - 2*xp2))/(2*((Y - a_yp)^2 + (Z - a_zp)^2 + (X - xp2)^2)^(3/2))))/(4*pi*((Y - a_yp)^2 + (Z - a_zp)^2));
dBy_dx = dByp_dx + dByn_dx;

dByp_dy = (I*Z*m0*(((X - xp1)*(2*Y - 2*a_yp))/(2*((Y - a_yp)^2 + (Z - a_zp)^2 + (X - xp1)^2)^(3/2)) - ((X - xp2)*(2*Y - 2*a_yp))/(2*((Y - a_yp)^2 + (Z - a_zp)^2 + (X - xp2)^2)^(3/2))))/(4*pi*((Y - a_yp)^2 + (Z - a_zp)^2)) + (I*Z*m0*(2*Y - 2*a_yp)*((X - xp1)/((Y - a_yp)^2 + (Z - a_zp)^2 + (X - xp1)^2)^(1/2) - (X - xp2)/((Y - a_yp)^2 + (Z - a_zp)^2 + (X - xp2)^2)^(1/2)))/(4*pi*((Y - a_yp)^2 + (Z - a_zp)^2)^2);
dByn_dy = - (I*Z*m0*(((X - xn1)*(2*Y - 2*a_yn))/(2*((Y - a_yn)^2 + (Z - a_zp)^2 + (X - xn1)^2)^(3/2)) - ((X - xn2)*(2*Y - 2*a_yn))/(2*((Y - a_yn)^2 + (Z - a_zp)^2 + (X - xn2)^2)^(3/2))))/(4*pi*((Y - a_yn)^2 + (Z - a_zp)^2)) - (I*Z*m0*(2*Y - 2*a_yn)*((X - xn1)/((Y - a_yn)^2 + (Z - a_zp)^2 + (X - xn1)^2)^(1/2) - (X - xn2)/((Y - a_yn)^2 + (Z - a_zp)^2 + (X - xn2)^2)^(1/2)))/(4*pi*((Y - a_yn)^2 + (Z - a_zp)^2)^2);
dBy_dy = dByp_dy + dByn_dy;

dByp_dz = (I*Z*m0*(((X - xp1)*(2*Z - 2*a_zp))/(2*((Y - a_yp)^2 + (Z - a_zp)^2 + (X - xp1)^2)^(3/2)) - ((X - xp2)*(2*Z - 2*a_zp))/(2*((Y - a_yp)^2 + (Z - a_zp)^2 + (X - xp2)^2)^(3/2))))/(4*pi*((Y - a_yp)^2 + (Z - a_zp)^2)) - (I*m0*((X - xp1)/((Y - a_yp)^2 + (Z - a_zp)^2 + (X - xp1)^2)^(1/2) - (X - xp2)/((Y - a_yp)^2 + (Z - a_zp)^2 + (X - xp2)^2)^(1/2)))/(4*pi*((Y - a_yp)^2 + (Z - a_zp)^2)) + (I*Z*m0*(2*Z - 2*a_zp)*((X - xp1)/((Y - a_yp)^2 + (Z - a_zp)^2 + (X - xp1)^2)^(1/2) - (X - xp2)/((Y - a_yp)^2 + (Z - a_zp)^2 + (X - xp2)^2)^(1/2)))/(4*pi*((Y - a_yp)^2 + (Z - a_zp)^2)^2);
dByn_dz = (I*m0*((X - xn1)/((Y - a_yn)^2 + (Z - a_zp)^2 + (X - xn1)^2)^(1/2) - (X - xn2)/((Y - a_yn)^2 + (Z - a_zp)^2 + (X - xn2)^2)^(1/2)))/(4*pi*((Y - a_yn)^2 + (Z - a_zp)^2)) - (I*Z*m0*(((X - xn1)*(2*Z - 2*a_zp))/(2*((Y - a_yn)^2 + (Z - a_zp)^2 + (X - xn1)^2)^(3/2)) - ((X - xn2)*(2*Z - 2*a_zp))/(2*((Y - a_yn)^2 + (Z - a_zp)^2 + (X - xn2)^2)^(3/2))))/(4*pi*((Y - a_yn)^2 + (Z - a_zp)^2)) - (I*Z*m0*(2*Z - 2*a_zp)*((X - xn1)/((Y - a_yn)^2 + (Z - a_zp)^2 + (X - xn1)^2)^(1/2) - (X - xn2)/((Y - a_yn)^2 + (Z - a_zp)^2 + (X - xn2)^2)^(1/2)))/(4*pi*((Y - a_yn)^2 + (Z - a_zp)^2)^2);
dBy_dz = dByp_dz + dByn_dz;

dBzp_dx = (I*m0*(Y - a_yp)*(1/((Y - a_yp)^2 + (Z - a_zp)^2 + (X - xp1)^2)^(1/2) - 1/((Y - a_yp)^2 + (Z - a_zp)^2 + (X - xp2)^2)^(1/2) - ((X - xp1)*(2*X - 2*xp1))/(2*((Y - a_yp)^2 + (Z - a_zp)^2 + (X - xp1)^2)^(3/2)) + ((X - xp2)*(2*X - 2*xp2))/(2*((Y - a_yp)^2 + (Z - a_zp)^2 + (X - xp2)^2)^(3/2))))/(4*pi*(Z^2 + (Y - a_yp)^2));
dBzn_dx = -(I*m0*(Y - a_yn)*(1/((Y - a_yn)^2 + (Z - a_zp)^2 + (X - xn1)^2)^(1/2) - 1/((Y - a_yn)^2 + (Z - a_zp)^2 + (X - xn2)^2)^(1/2) - ((X - xn1)*(2*X - 2*xn1))/(2*((Y - a_yn)^2 + (Z - a_zp)^2 + (X - xn1)^2)^(3/2)) + ((X - xn2)*(2*X - 2*xn2))/(2*((Y - a_yn)^2 + (Z - a_zp)^2 + (X - xn2)^2)^(3/2))))/(4*pi*(Z^2 + (Y - a_yn)^2));
dBz_dx = dBzp_dx + dBzn_dx;

dBzn_dy = (I*m0*(Y - a_yn)*(((X - xn1)*(2*Y - 2*a_yn))/(2*((Y - a_yn)^2 + (Z - a_zp)^2 + (X - xn1)^2)^(3/2)) - ((X - xn2)*(2*Y - 2*a_yn))/(2*((Y - a_yn)^2 + (Z - a_zp)^2 + (X - xn2)^2)^(3/2))))/(4*pi*(Z^2 + (Y - a_yn)^2)) - (I*m0*((X - xn1)/((Y - a_yn)^2 + (Z - a_zp)^2 + (X - xn1)^2)^(1/2) - (X - xn2)/((Y - a_yn)^2 + (Z - a_zp)^2 + (X - xn2)^2)^(1/2)))/(4*pi*(Z^2 + (Y - a_yn)^2)) + (I*m0*(Y - a_yn)*(2*Y - 2*a_yn)*((X - xn1)/((Y - a_yn)^2 + (Z - a_zp)^2 + (X - xn1)^2)^(1/2) - (X - xn2)/((Y - a_yn)^2 + (Z - a_zp)^2 + (X - xn2)^2)^(1/2)))/(4*pi*(Z^2 + (Y - a_yn)^2)^2);
dBzp_dy = (I*m0*((X - xp1)/((Y - a_yp)^2 + (Z - a_zp)^2 + (X - xp1)^2)^(1/2) - (X - xp2)/((Y - a_yp)^2 + (Z - a_zp)^2 + (X - xp2)^2)^(1/2)))/(4*pi*(Z^2 + (Y - a_yp)^2)) - (I*m0*(Y - a_yp)*(((X - xp1)*(2*Y - 2*a_yp))/(2*((Y - a_yp)^2 + (Z - a_zp)^2 + (X - xp1)^2)^(3/2)) - ((X - xp2)*(2*Y - 2*a_yp))/(2*((Y - a_yp)^2 + (Z - a_zp)^2 + (X - xp2)^2)^(3/2))))/(4*pi*(Z^2 + (Y - a_yp)^2)) - (I*m0*(Y - a_yp)*(2*Y - 2*a_yp)*((X - xp1)/((Y - a_yp)^2 + (Z - a_zp)^2 + (X - xp1)^2)^(1/2) - (X - xp2)/((Y - a_yp)^2 + (Z - a_zp)^2 + (X - xp2)^2)^(1/2)))/(4*pi*(Z^2 + (Y - a_yp)^2)^2);
dBz_dy = dBzn_dy + dBzp_dy;

dBzn_dz = (I*m0*(Y - a_yn)*(((X - xn1)*(2*Z - 2*a_zp))/(2*((Y - a_yn)^2 + (Z - a_zp)^2 + (X - xn1)^2)^(3/2)) - ((X - xn2)*(2*Z - 2*a_zp))/(2*((Y - a_yn)^2 + (Z - a_zp)^2 + (X - xn2)^2)^(3/2))))/(4*pi*(Z^2 + (Y - a_yn)^2)) + (I*Z*m0*(Y - a_yn)*((X - xn1)/((Y - a_yn)^2 + (Z - a_zp)^2 + (X - xn1)^2)^(1/2) - (X - xn2)/((Y - a_yn)^2 + (Z - a_zp)^2 + (X - xn2)^2)^(1/2)))/(2*pi*(Z^2 + (Y - a_yn)^2)^2);
dBzp_dz = - (I*m0*(Y - a_yp)*(((X - xp1)*(2*Z - 2*a_zp))/(2*((Y - a_yp)^2 + (Z - a_zp)^2 + (X - xp1)^2)^(3/2)) - ((X - xp2)*(2*Z - 2*a_zp))/(2*((Y - a_yp)^2 + (Z - a_zp)^2 + (X - xp2)^2)^(3/2))))/(4*pi*(Z^2 + (Y - a_yp)^2)) - (I*Z*m0*(Y - a_yp)*((X - xp1)/((Y - a_yp)^2 + (Z - a_zp)^2 + (X - xp1)^2)^(1/2) - (X - xp2)/((Y - a_yp)^2 + (Z - a_zp)^2 + (X - xp2)^2)^(1/2)))/(2*pi*(Z^2 + (Y - a_yp)^2)^2);
dBz_dz = dBzn_dz + dBzp_dz;
end

== matlab function latest_coil/Outer Coil/Coil 6/MATLAB Function3 ==
  data: X input; Hx_yp output; Y input; Z input; I input; Hy_yp output; Hz_yp output; Hx_yn output; Hy_yn output; Hz_yn output; dBx_dx output; dBx_dy output; dBx_dz output; dBz_dx output; dBz_dy output; dBz_dz output
function [Hx_yp, Hy_yp, Hz_yp, Hx_yn, Hy_yn, Hz_yn, dBx_dx, dBx_dy, dBx_dz, dBz_dx, dBz_dy, dBz_dz] = field_y(X, Y, Z, I)

n = 6;
gy = 420e-6;
% gx = 2.675e-3; 
gz = 0;
m0 = 4*pi*1e-7;
k = 0.4e-3;
yp1 = -0.6e-3 - (n-1)*k;
yp2 = 0.6e-3 + (n-1)*k;
a_xp = gy;
a_zp = gz;
k_yp = 1./(4*pi*((a_xp-X).^2+(a_zp-Z).^2));
kyp = (yp2-Y)./((yp2-Y).^2+(a_xp-X).^2+(a_zp-Z).^2).^0.5;
k_2yp = (yp1-Y)./((yp1-Y).^2+(a_xp-X).^2+(a_zp-Z).^2).^0.5;

Hx_yp = -((a_zp-Z).*k_yp.*(kyp - k_2yp))*I*m0;
Hy_yp = zeros(size(X,1),size(Y,1),size(Z,1));
Hz_yp = (-(a_xp-X).*k_yp.*(kyp - k_2yp))*I*m0;

a_xn = -gy;
yn1 = -0.8e-3 - (n-1)*k;
yn2 = 0.8e-3 + (n-1)*k;
k_yn = 1./(4*pi*((a_xn-X).^2+(a_zp-Z).^2));
kyn = (yn2-Y)./((yn2-Y).^2+(a_xn-X).^2+(a_zp-Z).^2).^0.5;
k_2yn = (yn1-Y)./((yn1-Y).^2+(a_xn-X).^2+(a_zp-Z).^2).^0.5;

Hx_yn = ((a_zp-Z).*k_yn.*(kyn - k_2yn))*I*m0;
Hy_yn = zeros(size(X,1),size(Y,1),size(Z,1));
Hz_yn = ((a_xn-X).*k_yn.*(kyn - k_2yn))*I*m0;

dBxn_dx = - (I*Z*m0*(((Y - yn1)*(2*X - 2*a_xn))/(2*((X - a_xn)^2 + (Z - a_zp)^2 + (Y - yn1)^2)^(3/2)) - ((Y - yn2)*(2*X - 2*a_xn))/(2*((X - a_xn)^2 + (Z - a_zp)^2 + (Y - yn2)^2)^(3/2))))/(4*pi*((X - a_xn)^2 + (Z - a_zp)^2)) - (I*Z*m0*((Y - yn1)/((X - a_xn)^2 + (Z - a_zp)^2 + (Y - yn1)^2)^(1/2) - (Y - yn2)/((X - a_xn)^2 + (Z - a_zp)^2 + (Y - yn2)^2)^(1/2))*(2*X - 2*a_xn))/(4*pi*((X - a_xn)^2 + (Z - a_zp)^2)^2);
dBxp_dx = (I*Z*m0*(((Y - yp1)*(2*X - 2*a_xp))/(2*((X - a_xp)^2 + (Z - a_zp)^2 + (Y - yp1)^2)^(3/2)) - ((Y - yp2)*(2*X - 2*a_xp))/(2*((X - a_xp)^2 + (Z - a_zp)^2 + (Y - yp2)^2)^(3/2))))/(4*pi*((X - a_xp)^2 + (Z - a_zp)^2)) + (I*Z*m0*((Y - yp1)/((X - a_xp)^2 + (Z - a_zp)^2 + (Y - yp1)^2)^(1/2) - (Y - yp2)/((X - a_xp)^2 + (Z - a_zp)^2 + (Y - yp2)^2)^(1/2))*(2*X - 2*a_xp))/(4*pi*((X - a_xp)^2 + (Z - a_zp)^2)^2);
dBx_dx = dBxp_dx + dBxn_dx;

dBxp_dy = -(I*Z*m0*(1/((X - a_xp)^2 + (Z - a_zp)^2 + (Y - yp1)^2)^(1/2) - 1/((X - a_xp)^2 + (Z - a_zp)^2 + (Y - yp2)^2)^(1/2) - ((Y - yp1)*(2*Y - 2*yp1))/(2*((X - a_xp)^2 + (Z - a_zp)^2 + (Y - yp1)^2)^(3/2)) + ((Y - yp2)*(2*Y - 2*yp2))/(2*((X - a_xp)^2 + (Z - a_zp)^2 + (Y - yp2)^2)^(3/2))))/(4*pi*((X - a_xp)^2 + (Z - a_zp)^2));
dBxn_dy = (I*Z*m0*(1/((X - a_xn)^2 + (Z - a_zp)^2 + (Y - yn1)^2)^(1/2) - 1/((X - a_xn)^2 + (Z - a_zp)^2 + (Y - yn2)^2)^(1/2) - ((Y - yn1)*(2*Y - 2*yn1))/(2*((X - a_xn)^2 + (Z - a_zp)^2 + (Y - yn1)^2)^(3/2)) + ((Y - yn2)*(2*Y - 2*yn2))/(2*((X - a_xn)^2 + (Z - a_zp)^2 + (Y - yn2)^2)^(3/2))))/(4*pi*((X - a_xn)^2 + (Z - a_zp)^2));
dBx_dy = dBxp_dy + dBxn_dy;

dBxp_dz = (I*Z*m0*(((Y - yp1)*(2*Z - 2*a_zp))/(2*((X - a_xp)^2 + (Z - a_zp)^2 + (Y - yp1)^2)^(3/2)) - ((Y - yp2)*(2*Z - 2*a_zp))/(2*((X - a_xp)^2 + (Z - a_zp)^2 + (Y - yp2)^2)^(3/2))))/(4*pi*((X - a_xp)^2 + (Z - a_zp)^2)) - (I*m0*((Y - yp1)/((X - a_xp)^2 + (Z - a_zp)^2 + (Y - yp1)^2)^(1/2) - (Y - yp2)/((X - a_xp)^2 + (Z - a_zp)^2 + (Y - yp2)^2)^(1/2)))/(4*pi*((X - a_xp)^2 + (Z - a_zp)^2)) + (I*Z*m0*((Y - yp1)/((X - a_xp)^2 + (Z - a_zp)^2 + (Y - yp1)^2)^(1/2) - (Y - yp2)/((X - a_xp)^2 + (Z - a_zp)^2 + (Y - yp2)^2)^(1/2))*(2*Z - 2*a_zp))/(4*pi*((X - a_xp)^2 + (Z - a_zp)^2)^2);
dBxn_dz = (I*m0*((Y - yn1)/((X - a_xn)^2 + (Z - a_zp)^2 + (Y - yn1)^2)^(1/2) - (Y - yn2)/((X - a_xn)^2 + (Z - a_zp)^2 + (Y - yn2)^2)^(1/2)))/(4*pi*((X - a_xn)^2 + (Z - a_zp)^2)) - (I*Z*m0*(((Y - yn1)*(2*Z - 2*a_zp))/(2*((X - a_xn)^2 + (Z - a_zp)^2 + (Y - yn1)^2)^(3/2)) - ((Y - yn2)*(2*Z - 2*a_zp))/(2*((X - a_xn)^2 + (Z - a_zp)^2 + (Y - yn2)^2)^(3/2))))/(4*pi*((X - a_xn)^2 + (Z - a_zp)^2)) - (I*Z*m0*((Y - yn1)/((X - a_xn)^2 + (Z - a_zp)^2 + (Y - yn1)^2)^(1/2) - (Y - yn2)/((X - a_xn)^2 + (Z - a_zp)^2 + (Y - yn2)^2)^(1/2))*(2*Z - 2*a_zp))/(4*pi*((X - a_xn)^2 + (Z - a_zp)^2)^2);
dBx_dz = dBxp_dz + dBxn_dz;

dBzn_dx = (I*m0*(X - a_xn)*(((Y - yn1)*(2*X - 2*a_xn))/(2*((X - a_xn)^2 + (Z - a_zp)^2 + (Y - yn1)^2)^(3/2)) - ((Y - yn2)*(2*X - 2*a_xn))/(2*((X - a_xn)^2 + (Z - a_zp)^2 + (Y - yn2)^2)^(3/2))))/(4*pi*(Z^2 + (X - a_xn)^2)) - (I*m0*((Y - yn1)/((X - a_xn)^2 + (Z - a_zp)^2 + (Y - yn1)^2)^(1/2) - (Y - yn2)/((X - a_xn)^2 + (Z - a_zp)^2 + (Y - yn2)^2)^(1/2)))/(4*pi*(Z^2 + (X - a_xn)^2)) + (I*m0*((Y - yn1)/((X - a_xn)^2 + (Z - a_zp)^2 + (Y - yn1)^2)^(1/2) - (Y - yn2)/((X - a_xn)^2 + (Z - a_zp)^2 + (Y - yn2)^2)^(1/2))*(X - a_xn)*(2*X - 2*a_xn))/(4*pi*(Z^2 + (X - a_xn)^2)^2);
dBzp_dx = (I*m0*((Y - yp1)/((X - a_xp)^2 + (Z - a_zp)^2 + (Y - yp1)^2)^(1/2) - (Y - yp2)/((X - a_xp)^2 + (Z - a_zp)^2 + (Y - yp2)^2)^(1/2)))/(4*pi*(Z^2 + (X - a_xp)^2)) - (I*m0*(X - a_xp)*(((Y - yp1)*(2*X - 2*a_xp))/(2*((X - a_xp)^2 + (Z - a_zp)^2 + (Y - yp1)^2)^(3/2)) - ((Y - yp2)*(2*X - 2*a_xp))/(2*((X - a_xp)^2 + (Z - a_zp)^2 + (Y - yp2)^2)^(3/2))))/(4*pi*(Z^2 + (X - a_xp)^2)) - (I*m0*((Y - yp1)/((X - a_xp)^2 + (Z - a_zp)^2 + (Y - yp1)^2)^(1/2) - (Y - yp2)/((X - a_xp)^2 + (Z - a_zp)^2 + (Y - yp2)^2)^(1/2))*(X - a_xp)*(2*X - 2*a_xp))/(4*pi*(Z^2 + (X - a_xp)^2)^2);
dBz_dx = dBzp_dx + dBzn_dx;

dBzn_dy = -(I*m0*(X - a_xn)*(1/((X - a_xn)^2 + (Z - a_zp)^2 + (Y - yn1)^2)^(1/2) - 1/((X - a_xn)^2 + (Z - a_zp)^2 + (Y - yn2)^2)^(1/2) - ((Y - yn1)*(2*Y - 2*yn1))/(2*((X - a_xn)^2 + (Z - a_zp)^2 + (Y - yn1)^2)^(3/2)) + ((Y - yn2)*(2*Y - 2*yn2))/(2*((X - a_xn)^2 + (Z - a_zp)^2 + (Y - yn2)^2)^(3/2))))/(4*pi*(Z^2 + (X - a_xn)^2));
dBzp_dy = (I*m0*(X - a_xp)*(1/((X - a_xp)^2 + (Z - a_zp)^2 + (Y - yp1)^2)^(1/2) - 1/((X - a_xp)^2 + (Z - a_zp)^2 + (Y - yp2)^2)^(1/2) - ((Y - yp1)*(2*Y - 2*yp1))/(2*((X - a_xp)^2 + (Z - a_zp)^2 + (Y - yp1)^2)^(3/2)) + ((Y - yp2)*(2*Y - 2*yp2))/(2*((X - a_xp)^2 + (Z - a_zp)^2 + (Y - yp2)^2)^(3/2))))/(4*pi*(Z^2 + (X - a_xp)^2));
dBz_dy = dBzn_dy + dBzp_dy;

dBzn_dz = (I*m0*(X - a_xn)*(((Y - yn1)*(2*Z - 2*a_zp))/(2*((X - a_xn)^2 + (Z - a_zp)^2 + (Y - yn1)^2)^(3/2)) - ((Y - yn2)*(2*Z - 2*a_zp))/(2*((X - a_xn)^2 + (Z - a_zp)^2 + (Y - yn2)^2)^(3/2))))/(4*pi*(Z^2 + (X - a_xn)^2)) + (I*Z*m0*((Y - yn1)/((X - a_xn)^2 + (Z - a_zp)^2 + (Y - yn1)^2)^(1/2) - (Y - yn2)/((X - a_xn)^2 + (Z - a_zp)^2 + (Y - yn2)^2)^(1/2))*(X - a_xn))/(2*pi*(Z^2 + (X - a_xn)^2)^2);
dBzp_dz = - (I*m0*(X - a_xp)*(((Y - yp1)*(2*Z - 2*a_zp))/(2*((X - a_xp)^2 + (Z - a_zp)^2 + (Y - yp1)^2)^(3/2)) - ((Y - yp2)*(2*Z - 2*a_zp))/(2*((X - a_xp)^2 + (Z - a_zp)^2 + (Y - yp2)^2)^(3/2))))/(4*pi*(Z^2 + (X - a_xp)^2)) - (I*Z*m0*((Y - yp1)/((X - a_xp)^2 + (Z - a_zp)^2 + (Y - yp1)^2)^(1/2) - (Y - yp2)/((X - a_xp)^2 + (Z - a_zp)^2 + (Y - yp2)^2)^(1/2))*(X - a_xp))/(2*pi*(Z^2 + (X - a_xp)^2)^2);
dBz_dz = dBzn_dz + dBzp_dz;
end

== matlab function latest_coil/Outer Coil/Coil 6/MATLAB Function4 ==
  data: Hx_xp input; Hy_xp input; Hz_xp input; Hx output; Hx_xn input; Hy_xn input; Hy output; Hz output; Hz_xn input; Hx_yp input; Hy_yp input; Hz_yp input; Hx_yn input; Hy_yn input; Hz_yn input
function [Hx, Hy, Hz] = field_sum(Hx_xp, Hy_xp, Hz_xp, Hx_xn, Hy_xn, Hz_xn, Hx_yp, Hy_yp, Hz_yp, Hx_yn, Hy_yn, Hz_yn)
Hx = Hx_xp + Hx_xn + Hx_yp + Hx_yn;
Hy = Hy_xp + Hy_xn + Hy_yp + Hy_yn;
Hz = Hz_xp + Hz_xn + Hz_yp + Hz_yn;
end

== matlab function latest_coil/Outer Coil/Coil 7/MATLAB Function ==
  data: X input; Hx_xp output; Y input; Z input; I input; Hy_xp output; Hz_xp output; Hx_xn output; Hy_xn output; Hz_xn output; dBy_dx output; dBy_dy output; dBy_dz output; dBz_dx output; dBz_dy output; dBz_dz output
function [Hx_xp, Hy_xp, Hz_xp, Hx_xn, Hy_xn, Hz_xn,dBy_dx ,dBy_dy, dBy_dz, dBz_dx ,dBz_dy, dBz_dz] = field_x(X, Y, Z, I)
n = 7;
% gy = 417.14e-6; 
gx = 3.075e-3; 
gz = 0;
m0 = 4*pi*1e-7;
k = 0.4e-3;
xp1 = -0.8e-3 - (n-1)*k;
xp2 = 0.8e-3 + (n-1)*k;
a_yp = gx; 
a_zp = gz;
k_p = 1./(4*pi*((a_yp-Y).^2+(a_zp-Z).^2));
kxp = (xp2-X)./((xp2-X).^2+(a_yp-Y).^2+(a_zp-Z).^2).^0.5;
k_2xp = (xp1-X)./((xp1-X).^2+(a_yp-Y).^2+(a_zp-Z).^2).^0.5;

Hx_xp = zeros(size(X,1),size(Y,1),size(Z,1));
Hy_xp = (-(a_zp-Z).*k_p.*(kxp - k_2xp))*I*m0;
Hz_xp = (-(a_yp-Y).*k_p.*(kxp - k_2xp))*I*m0;

a_yn = -gx;
xn1 = -1e-3 - (n-1)*k;
xn2 = 1e-3 + (n-1)*k;
k_n = 1./(4*pi*((a_yn-Y).^2+(a_zp-Z).^2));
kxn = (xn2-X)./((xn2-X).^2+(a_yn-Y).^2+(a_zp-Z).^2).^0.5;
k_2xn = (xn1-X)./((xn1-X).^2+(a_yn-Y).^2+(a_zp-Z).^2).^0.5;

Hx_xn = zeros(size(X,1),size(Y,1),size(Z,1));
Hy_xn = ((a_zp-Z).*k_n.*(kxn - k_2xn))*I*m0;
Hz_xn = ((a_yn-Y).*k_n.*(kxn - k_2xn))*I*m0;

dByn_dx = (I*Z*m0*(1/((Y - a_yn)^2 + (Z - a_zp)^2 + (X - xn1)^2)^(1/2) - 1/((Y - a_yn)^2 + (Z - a_zp)^2 + (X - xn2)^2)^(1/2) - ((X - xn1)*(2*X - 2*xn1))/(2*((Y - a_yn)^2 + (Z - a_zp)^2 + (X - xn1)^2)^(3/2)) + ((X - xn2)*(2*X - 2*xn2))/(2*((Y - a_yn)^2 + (Z - a_zp)^2 + (X - xn2)^2)^(3/2))))/(4*pi*((Y - a_yn)^2 + (Z - a_zp)^2));
dByp_dx = -(I*Z*m0*(1/((Y - a_yp)^2 + (Z - a_zp)^2 + (X - xp1)^2)^(1/2) - 1/((Y - a_yp)^2 + (Z - a_zp)^2 + (X - xp2)^2)^(1/2) - ((X - xp1)*(2*X - 2*xp1))/(2*((Y - a_yp)^2 + (Z - a_zp)^2 + (X - xp1)^2)^(3/2)) + ((X - xp2)*(2*X - 2*xp2))/(2*((Y - a_yp)^2 + (Z - a_zp)^2 + (X - xp2)^2)^(3/2))))/(4*pi*((Y - a_yp)^2 + (Z - a_zp)^2));
dBy_dx = dByp_dx + dByn_dx;

dByp_dy = (I*Z*m0*(((X - xp1)*(2*Y - 2*a_yp))/(2*((Y - a_yp)^2 + (Z - a_zp)^2 + (X - xp1)^2)^(3/2)) - ((X - xp2)*(2*Y - 2*a_yp))/(2*((Y - a_yp)^2 + (Z - a_zp)^2 + (X - xp2)^2)^(3/2))))/(4*pi*((Y - a_yp)^2 + (Z - a_zp)^2)) + (I*Z*m0*(2*Y - 2*a_yp)*((X - xp1)/((Y - a_yp)^2 + (Z - a_zp)^2 + (X - xp1)^2)^(1/2) - (X - xp2)/((Y - a_yp)^2 + (Z - a_zp)^2 + (X - xp2)^2)^(1/2)))/(4*pi*((Y - a_yp)^2 + (Z - a_zp)^2)^2);
dByn_dy = - (I*Z*m0*(((X - xn1)*(2*Y - 2*a_yn))/(2*((Y - a_yn)^2 + (Z - a_zp)^2 + (X - xn1)^2)^(3/2)) - ((X - xn2)*(2*Y - 2*a_yn))/(2*((Y - a_yn)^2 + (Z - a_zp)^2 + (X - xn2)^2)^(3/2))))/(4*pi*((Y - a_yn)^2 + (Z - a_zp)^2)) - (I*Z*m0*(2*Y - 2*a_yn)*((X - xn1)/((Y - a_yn)^2 + (Z - a_zp)^2 + (X - xn1)^2)^(1/2) - (X - xn2)/((Y - a_yn)^2 + (Z - a_zp)^2 + (X - xn2)^2)^(1/2)))/(4*pi*((Y - a_yn)^2 + (Z - a_zp)^2)^2);
dBy_dy = dByp_dy + dByn_dy;

dByp_dz = (I*Z*m0*(((X - xp1)*(2*Z - 2*a_zp))/(2*((Y - a_yp)^2 + (Z - a_zp)^2 + (X - xp1)^2)^(3/2)) - ((X - xp2)*(2*Z - 2*a_zp))/(2*((Y - a_yp)^2 + (Z - a_zp)^2 + (X - xp2)^2)^(3/2))))/(4*pi*((Y - a_yp)^2 + (Z - a_zp)^2)) - (I*m0*((X - xp1)/((Y - a_yp)^2 + (Z - a_zp)^2 + (X - xp1)^2)^(1/2) - (X - xp2)/((Y - a_yp)^2 + (Z - a_zp)^2 + (X - xp2)^2)^(1/2)))/(4*pi*((Y - a_yp)^2 + (Z - a_zp)^2)) + (I*Z*m0*(2*Z - 2*a_zp)*((X - xp1)/((Y - a_yp)^2 + (Z - a_zp)^2 + (X - xp1)^2)^(1/2) - (X - xp2)/((Y - a_yp)^2 + (Z - a_zp)^2 + (X - xp2)^2)^(1/2)))/(4*pi*((Y - a_yp)^2 + (Z - a_zp)^2)^2);
dByn_dz = (I*m0*((X - xn1)/((Y - a_yn)^2 + (Z - a_zp)^2 + (X - xn1)^2)^(1/2) - (X - xn2)/((Y - a_yn)^2 + (Z - a_zp)^2 + (X - xn2)^2)^(1/2)))/(4*pi*((Y - a_yn)^2 + (Z - a_zp)^2)) - (I*Z*m0*(((X - xn1)*(2*Z - 2*a_zp))/(2*((Y - a_yn)^2 + (Z - a_zp)^2 + (X - xn1)^2)^(3/2)) - ((X - xn2)*(2*Z - 2*a_zp))/(2*((Y - a_yn)^2 + (Z - a_zp)^2 + (X - xn2)^2)^(3/2))))/(4*pi*((Y - a_yn)^2 + (Z - a_zp)^2)) - (I*Z*m0*(2*Z - 2*a_zp)*((X - xn1)/((Y - a_yn)^2 + (Z - a_zp)^2 + (X - xn1)^2)^(1/2) - (X - xn2)/((Y - a_yn)^2 + (Z - a_zp)^2 + (X - xn2)^2)^(1/2)))/(4*pi*((Y - a_yn)^2 + (Z - a_zp)^2)^2);
dBy_dz = dByp_dz + dByn_dz;

dBzp_dx = (I*m0*(Y - a_yp)*(1/((Y - a_yp)^2 + (Z - a_zp)^2 + (X - xp1)^2)^(1/2) - 1/((Y - a_yp)^2 + (Z - a_zp)^2 + (X - xp2)^2)^(1/2) - ((X - xp1)*(2*X - 2*xp1))/(2*((Y - a_yp)^2 + (Z - a_zp)^2 + (X - xp1)^2)^(3/2)) + ((X - xp2)*(2*X - 2*xp2))/(2*((Y - a_yp)^2 + (Z - a_zp)^2 + (X - xp2)^2)^(3/2))))/(4*pi*(Z^2 + (Y - a_yp)^2));
dBzn_dx = -(I*m0*(Y - a_yn)*(1/((Y - a_yn)^2 + (Z - a_zp)^2 + (X - xn1)^2)^(1/2) - 1/((Y - a_yn)^2 + (Z - a_zp)^2 + (X - xn2)^2)^(1/2) - ((X - xn1)*(2*X - 2*xn1))/(2*((Y - a_yn)^2 + (Z - a_zp)^2 + (X - xn1)^2)^(3/2)) + ((X - xn2)*(2*X - 2*xn2))/(2*((Y - a_yn)^2 + (Z - a_zp)^2 + (X - xn2)^2)^(3/2))))/(4*pi*(Z^2 + (Y - a_yn)^2));
dBz_dx = dBzp_dx + dBzn_dx;

dBzn_dy = (I*m0*(Y - a_yn)*(((X - xn1)*(2*Y - 2*a_yn))/(2*((Y - a_yn)^2 + (Z - a_zp)^2 + (X - xn1)^2)^(3/2)) - ((X - xn2)*(2*Y - 2*a_yn))/(2*((Y - a_yn)^2 + (Z - a_zp)^2 + (X - xn2)^2)^(3/2))))/(4*pi*(Z^2 + (Y - a_yn)^2)) - (I*m0*((X - xn1)/((Y - a_yn)^2 + (Z - a_zp)^2 + (X - xn1)^2)^(1/2) - (X - xn2)/((Y - a_yn)^2 + (Z - a_zp)^2 + (X - xn2)^2)^(1/2)))/(4*pi*(Z^2 + (Y - a_yn)^2)) + (I*m0*(Y - a_yn)*(2*Y - 2*a_yn)*((X - xn1)/((Y - a_yn)^2 + (Z - a_zp)^2 + (X - xn1)^2)^(1/2) - (X - xn2)/((Y - a_yn)^2 + (Z - a_zp)^2 + (X - xn2)^2)^(1/2)))/(4*pi*(Z^2 + (Y - a_yn)^2)^2);
dBzp_dy = (I*m0*((X - xp1)/((Y - a_yp)^2 + (Z - a_zp)^2 + (X - xp1)^2)^(1/2) - (X - xp2)/((Y - a_yp)^2 + (Z - a_zp)^2 + (X - xp2)^2)^(1/2)))/(4*pi*(Z^2 + (Y - a_yp)^2)) - (I*m0*(Y - a_yp)*(((X - xp1)*(2*Y - 2*a_yp))/(2*((Y - a_yp)^2 + (Z - a_zp)^2 + (X - xp1)^2)^(3/2)) - ((X - xp2)*(2*Y - 2*a_yp))/(2*((Y - a_yp)^2 + (Z - a_zp)^2 + (X - xp2)^2)^(3/2))))/(4*pi*(Z^2 + (Y - a_yp)^2)) - (I*m0*(Y - a_yp)*(2*Y - 2*a_yp)*((X - xp1)/((Y - a_yp)^2 + (Z - a_zp)^2 + (X - xp1)^2)^(1/2) - (X - xp2)/((Y - a_yp)^2 + (Z - a_zp)^2 + (X - xp2)^2)^(1/2)))/(4*pi*(Z^2 + (Y - a_yp)^2)^2);
dBz_dy = dBzn_dy + dBzp_dy;

dBzn_dz = (I*m0*(Y - a_yn)*(((X - xn1)*(2*Z - 2*a_zp))/(2*((Y - a_yn)^2 + (Z - a_zp)^2 + (X - xn1)^2)^(3/2)) - ((X - xn2)*(2*Z - 2*a_zp))/(2*((Y - a_yn)^2 + (Z - a_zp)^2 + (X - xn2)^2)^(3/2))))/(4*pi*(Z^2 + (Y - a_yn)^2)) + (I*Z*m0*(Y - a_yn)*((X - xn1)/((Y - a_yn)^2 + (Z - a_zp)^2 + (X - xn1)^2)^(1/2) - (X - xn2)/((Y - a_yn)^2 + (Z - a_zp)^2 + (X - xn2)^2)^(1/2)))/(2*pi*(Z^2 + (Y - a_yn)^2)^2);
dBzp_dz = - (I*m0*(Y - a_yp)*(((X - xp1)*(2*Z - 2*a_zp))/(2*((Y - a_yp)^2 + (Z - a_zp)^2 + (X - xp1)^2)^(3/2)) - ((X - xp2)*(2*Z - 2*a_zp))/(2*((Y - a_yp)^2 + (Z - a_zp)^2 + (X - xp2)^2)^(3/2))))/(4*pi*(Z^2 + (Y - a_yp)^2)) - (I*Z*m0*(Y - a_yp)*((X - xp1)/((Y - a_yp)^2 + (Z - a_zp)^2 + (X - xp1)^2)^(1/2) - (X - xp2)/((Y - a_yp)^2 + (Z - a_zp)^2 + (X - xp2)^2)^(1/2)))/(2*pi*(Z^2 + (Y - a_yp)^2)^2);
dBz_dz = dBzn_dz + dBzp_dz;

end

== matlab function latest_coil/Outer Coil/Coil 7/MATLAB Function3 ==
  data: X input; Hx_yp output; Y input; Z input; I input; Hy_yp output; Hz_yp output; Hx_yn output; Hy_yn output; Hz_yn output; dBx_dx output; dBx_dy output; dBx_dz output; dBz_dx output; dBz_dy output; dBz_dz output
function [Hx_yp, Hy_yp, Hz_yp, Hx_yn, Hy_yn, Hz_yn, dBx_dx, dBx_dy, dBx_dz, dBz_dx, dBz_dy, dBz_dz] = field_y(X, Y, Z, I)

n = 7;
gy = 417.14e-6; 
% gx = 3.075e-3; 
gz = 0;

m0 = 4*pi*1e-7;
k = 0.4e-3;
yp1 = -0.6e-3 - (n-1)*k;
yp2 = 0.6e-3 + (n-1)*k;
a_xp = gy;
a_zp = gz;
k_yp = 1./(4*pi*((a_xp-X).^2+(a_zp-Z).^2));
kyp = (yp2-Y)./((yp2-Y).^2+(a_xp-X).^2+(a_zp-Z).^2).^0.5;
k_2yp = (yp1-Y)./((yp1-Y).^2+(a_xp-X).^2+(a_zp-Z).^2).^0.5;

Hx_yp = -((a_zp-Z).*k_yp.*(kyp - k_2yp))*I*m0;
Hy_yp = zeros(size(X,1),size(Y,1),size(Z,1));
Hz_yp = (-(a_xp-X).*k_yp.*(kyp - k_2yp))*I*m0;

a_xn = -gy;
yn1 = -0.8e-3 - (n-1)*k;
yn2 = 0.8e-3 + (n-1)*k;
k_yn = 1./(4*pi*((a_xn-X).^2+(a_zp-Z).^2));
kyn = (yn2-Y)./((yn2-Y).^2+(a_xn-X).^2+(a_zp-Z).^2).^0.5;
k_2yn = (yn1-Y)./((yn1-Y).^2+(a_xn-X).^2+(a_zp-Z).^2).^0.5;

Hx_yn = ((a_zp-Z).*k_yn.*(kyn - k_2yn))*I*m0;
Hy_yn = zeros(size(X,1),size(Y,1),size(Z,1));
Hz_yn = ((a_xn-X).*k_yn.*(kyn - k_2yn))*I*m0;

dBxn_dx = - (I*Z*m0*(((Y - yn1)*(2*X - 2*a_xn))/(2*((X - a_xn)^2 + (Z - a_zp)^2 + (Y - yn1)^2)^(3/2)) - ((Y - yn2)*(2*X - 2*a_xn))/(2*((X - a_xn)^2 + (Z - a_zp)^2 + (Y - yn2)^2)^(3/2))))/(4*pi*((X - a_xn)^2 + (Z - a_zp)^2)) - (I*Z*m0*((Y - yn1)/((X - a_xn)^2 + (Z - a_zp)^2 + (Y - yn1)^2)^(1/2) - (Y - yn2)/((X - a_xn)^2 + (Z - a_zp)^2 + (Y - yn2)^2)^(1/2))*(2*X - 2*a_xn))/(4*pi*((X - a_xn)^2 + (Z - a_zp)^2)^2);
dBxp_dx = (I*Z*m0*(((Y - yp1)*(2*X - 2*a_xp))/(2*((X - a_xp)^2 + (Z - a_zp)^2 + (Y - yp1)^2)^(3/2)) - ((Y - yp2)*(2*X - 2*a_xp))/(2*((X - a_xp)^2 + (Z - a_zp)^2 + (Y - yp2)^2)^(3/2))))/(4*pi*((X - a_xp)^2 + (Z - a_zp)^2)) + (I*Z*m0*((Y - yp1)/((X - a_xp)^2 + (Z - a_zp)^2 + (Y - yp1)^2)^(1/2) - (Y - yp2)/((X - a_xp)^2 + (Z - a_zp)^2 + (Y - yp2)^2)^(1/2))*(2*X - 2*a_xp))/(4*pi*((X - a_xp)^2 + (Z - a_zp)^2)^2);
dBx_dx = dBxp_dx + dBxn_dx;

dBxp_dy = -(I*Z*m0*(1/((X - a_xp)^2 + (Z - a_zp)^2 + (Y - yp1)^2)^(1/2) - 1/((X - a_xp)^2 + (Z - a_zp)^2 + (Y - yp2)^2)^(1/2) - ((Y - yp1)*(2*Y - 2*yp1))/(2*((X - a_xp)^2 + (Z - a_zp)^2 + (Y - yp1)^2)^(3/2)) + ((Y - yp2)*(2*Y - 2*yp2))/(2*((X - a_xp)^2 + (Z - a_zp)^2 + (Y - yp2)^2)^(3/2))))/(4*pi*((X - a_xp)^2 + (Z - a_zp)^2));
dBxn_dy = (I*Z*m0*(1/((X - a_xn)^2 + (Z - a_zp)^2 + (Y - yn1)^2)^(1/2) - 1/((X - a_xn)^2 + (Z - a_zp)^2 + (Y - yn2)^2)^(1/2) - ((Y - yn1)*(2*Y - 2*yn1))/(2*((X - a_xn)^2 + (Z - a_zp)^2 + (Y - yn1)^2)^(3/2)) + ((Y - yn2)*(2*Y - 2*yn2))/(2*((X - a_xn)^2 + (Z - a_zp)^2 + (Y - yn2)^2)^(3/2))))/(4*pi*((X - a_xn)^2 + (Z - a_zp)^2));
dBx_dy = dBxp_dy + dBxn_dy;

dBxp_dz = (I*Z*m0*(((Y - yp1)*(2*Z - 2*a_zp))/(2*((X - a_xp)^2 + (Z - a_zp)^2 + (Y - yp1)^2)^(3/2)) - ((Y - yp2)*(2*Z - 2*a_zp))/(2*((X - a_xp)^2 + (Z - a_zp)^2 + (Y - yp2)^2)^(3/2))))/(4*pi*((X - a_xp)^2 + (Z - a_zp)^2)) - (I*m0*((Y - yp1)/((X - a_xp)^2 + (Z - a_zp)^2 + (Y - yp1)^2)^(1/2) - (Y - yp2)/((X - a_xp)^2 + (Z - a_zp)^2 + (Y - yp2)^2)^(1/2)))/(4*pi*((X - a_xp)^2 + (Z - a_zp)^2)) + (I*Z*m0*((Y - yp1)/((X - a_xp)^2 + (Z - a_zp)^2 + (Y - yp1)^2)^(1/2) - (Y - yp2)/((X - a_xp)^2 + (Z - a_zp)^2 + (Y - yp2)^2)^(1/2))*(2*Z - 2*a_zp))/(4*pi*((X - a_xp)^2 + (Z - a_zp)^2)^2);
dBxn_dz = (I*m0*((Y - yn1)/((X - a_xn)^2 + (Z - a_zp)^2 + (Y - yn1)^2)^(1/2) - (Y - yn2)/((X - a_xn)^2 + (Z - a_zp)^2 + (Y - yn2)^2)^(1/2)))/(4*pi*((X - a_xn)^2 + (Z - a_zp)^2)) - (I*Z*m0*(((Y - yn1)*(2*Z - 2*a_zp))/(2*((X - a_xn)^2 + (Z - a_zp)^2 + (Y - yn1)^2)^(3/2)) - ((Y - yn2)*(2*Z - 2*a_zp))/(2*((X - a_xn)^2 + (Z - a_zp)^2 + (Y - yn2)^2)^(3/2))))/(4*pi*((X - a_xn)^2 + (Z - a_zp)^2)) - (I*Z*m0*((Y - yn1)/((X - a_xn)^2 + (Z - a_zp)^2 + (Y - yn1)^2)^(1/2) - (Y - yn2)/((X - a_xn)^2 + (Z - a_zp)^2 + (Y - yn2)^2)^(1/2))*(2*Z - 2*a_zp))/(4*pi*((X - a_xn)^2 + (Z - a_zp)^2)^2);
dBx_dz = dBxp_dz + dBxn_dz;

dBzn_dx = (I*m0*(X - a_xn)*(((Y - yn1)*(2*X - 2*a_xn))/(2*((X - a_xn)^2 + (Z - a_zp)^2 + (Y - yn1)^2)^(3/2)) - ((Y - yn2)*(2*X - 2*a_xn))/(2*((X - a_xn)^2 + (Z - a_zp)^2 + (Y - yn2)^2)^(3/2))))/(4*pi*(Z^2 + (X - a_xn)^2)) - (I*m0*((Y - yn1)/((X - a_xn)^2 + (Z - a_zp)^2 + (Y - yn1)^2)^(1/2) - (Y - yn2)/((X - a_xn)^2 + (Z - a_zp)^2 + (Y - yn2)^2)^(1/2)))/(4*pi*(Z^2 + (X - a_xn)^2)) + (I*m0*((Y - yn1)/((X - a_xn)^2 + (Z - a_zp)^2 + (Y - yn1)^2)^(1/2) - (Y - yn2)/((X - a_xn)^2 + (Z - a_zp)^2 + (Y - yn2)^2)^(1/2))*(X - a_xn)*(2*X - 2*a_xn))/(4*pi*(Z^2 + (X - a_xn)^2)^2);
dBzp_dx = (I*m0*((Y - yp1)/((X - a_xp)^2 + (Z - a_zp)^2 + (Y - yp1)^2)^(1/2) - (Y - yp2)/((X - a_xp)^2 + (Z - a_zp)^2 + (Y - yp2)^2)^(1/2)))/(4*pi*(Z^2 + (X - a_xp)^2)) - (I*m0*(X - a_xp)*(((Y - yp1)*(2*X - 2*a_xp))/(2*((X - a_xp)^2 + (Z - a_zp)^2 + (Y - yp1)^2)^(3/2)) - ((Y - yp2)*(2*X - 2*a_xp))/(2*((X - a_xp)^2 + (Z - a_zp)^2 + (Y - yp2)^2)^(3/2))))/(4*pi*(Z^2 + (X - a_xp)^2)) - (I*m0*((Y - yp1)/((X - a_xp)^2 + (Z - a_zp)^2 + (Y - yp1)^2)^(1/2) - (Y - yp2)/((X - a_xp)^2 + (Z - a_zp)^2 + (Y - yp2)^2)^(1/2))*(X - a_xp)*(2*X - 2*a_xp))/(4*pi*(Z^2 + (X - a_xp)^2)^2);
dBz_dx = dBzp_dx + dBzn_dx;

dBzn_dy = -(I*m0*(X - a_xn)*(1/((X - a_xn)^2 + (Z - a_zp)^2 + (Y - yn1)^2)^(1/2) - 1/((X - a_xn)^2 + (Z - a_zp)^2 + (Y - yn2)^2)^(1/2) - ((Y - yn1)*(2*Y - 2*yn1))/(2*((X - a_xn)^2 + (Z - a_zp)^2 + (Y - yn1)^2)^(3/2)) + ((Y - yn2)*(2*Y - 2*yn2))/(2*((X - a_xn)^2 + (Z - a_zp)^2 + (Y - yn2)^2)^(3/2))))/(4*pi*(Z^2 + (X - a_xn)^2));
dBzp_dy = (I*m0*(X - a_xp)*(1/((X - a_xp)^2 + (Z - a_zp)^2 + (Y - yp1)^2)^(1/2) - 1/((X - a_xp)^2 + (Z - a_zp)^2 + (Y - yp2)^2)^(1/2) - ((Y - yp1)*(2*Y - 2*yp1))/(2*((X - a_xp)^2 + (Z - a_zp)^2 + (Y - yp1)^2)^(3/2)) + ((Y - yp2)*(2*Y - 2*yp2))/(2*((X - a_xp)^2 + (Z - a_zp)^2 + (Y - yp2)^2)^(3/2))))/(4*pi*(Z^2 + (X - a_xp)^2));
dBz_dy = dBzn_dy + dBzp_dy;

dBzn_dz = (I*m0*(X - a_xn)*(((Y - yn1)*(2*Z - 2*a_zp))/(2*((X - a_xn)^2 + (Z - a_zp)^2 + (Y - yn1)^2)^(3/2)) - ((Y - yn2)*(2*Z - 2*a_zp))/(2*((X - a_xn)^2 + (Z - a_zp)^2 + (Y - yn2)^2)^(3/2))))/(4*pi*(Z^2 + (X - a_xn)^2)) + (I*Z*m0*((Y - yn1)/((X - a_xn)^2 + (Z - a_zp)^2 + (Y - yn1)^2)^(1/2) - (Y - yn2)/((X - a_xn)^2 + (Z - a_zp)^2 + (Y - yn2)^2)^(1/2))*(X - a_xn))/(2*pi*(Z^2 + (X - a_xn)^2)^2);
dBzp_dz = - (I*m0*(X - a_xp)*(((Y - yp1)*(2*Z - 2*a_zp))/(2*((X - a_xp)^2 + (Z - a_zp)^2 + (Y - yp1)^2)^(3/2)) - ((Y - yp2)*(2*Z - 2*a_zp))/(2*((X - a_xp)^2 + (Z - a_zp)^2 + (Y - yp2)^2)^(3/2))))/(4*pi*(Z^2 + (X - a_xp)^2)) - (I*Z*m0*((Y - yp1)/((X - a_xp)^2 + (Z - a_zp)^2 + (Y - yp1)^2)^(1/2) - (Y - yp2)/((X - a_xp)^2 + (Z - a_zp)^2 + (Y - yp2)^2)^(1/2))*(X - a_xp))/(2*pi*(Z^2 + (X - a_xp)^2)^2);
dBz_dz = dBzn_dz + dBzp_dz;
end

== matlab function latest_coil/Outer Coil/Coil 7/MATLAB Function4 ==
  data: Hx_xp input; Hy_xp input; Hz_xp input; Hx output; Hx_xn input; Hy_xn input; Hy output; Hz output; Hz_xn input; Hx_yp input; Hy_yp input; Hz_yp input; Hx_yn input; Hy_yn input; Hz_yn input
function [Hx, Hy, Hz] = field_sum(Hx_xp, Hy_xp, Hz_xp, Hx_xn, Hy_xn, Hz_xn, Hx_yp, Hy_yp, Hz_yp, Hx_yn, Hy_yn, Hz_yn)
Hx = Hx_xp + Hx_xn + Hx_yp + Hx_yn;
Hy = Hy_xp + Hy_xn + Hy_yp + Hy_yn;
Hz = Hz_xp + Hz_xn + Hz_yp + Hz_yn;
end
